simulink model "Casa"  (R2017a)
settings: Solver=ode45  StartTime=0.0  StopTime=5.0  RelTol=1e-3  EnableMultiTasking=on
libraries: simulink x3
settings Model: Creator=LAB1-8  LastModifiedBy=Oscar
settings DataIOCC: LimitDataPoints=on  SaveFormat=Array
settings OptimizationCC: LifeSpan=inf
settings DebuggingCC: UnderspecifiedInitializationDetection=Classic  MergeDetectMultiDrivingBlocksExec=none  SolverPrmCheckMsg=warning  SFUnexpectedBacktrackingDiag=warning  SFNoUnconditionalDefaultTransitionDiag=warning  SFExecutionAtInitializationDiag=none
settings HardwareCC: ProdBitPerPointer=32  ProdBitPerSizeT=32  ProdBitPerPtrDiffT=32  ProdLargestAtomicFloat=None  ProdIntDivRoundTo=Undefined  ProdEndianess=Unspecified  ProdWordSize=32  ProdHWDeviceType=32-bit Generic
settings ModelReferenceCC: PropagateSignalLabelsOutOfModel=off
settings GRTTargetCC: TargetLangStandard=C89/C90 (ANSI)  GeneratePreprocessorConditionals=Disable all
settings ConfigComp: CovMetricSettings=dw  CovHtmlReporting=on  CovSaveCumulativeToWorkspaceVar=on  CovSaveSingleToWorkspaceVar=on  CovExternalEMLEnable=off

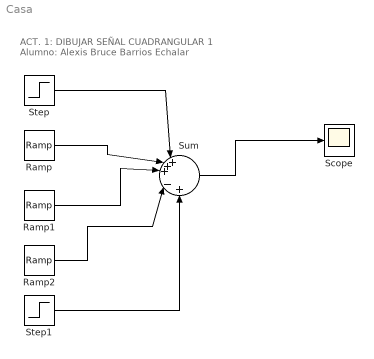
== system Casa ==
  note: ACT. 1: DIBUJAR SEÑAL CUADRANGULAR 1
      | Alumno: Alexis Bruce Barrios Echalar
  Ramp : simulink/Sources/Ramp  slope=1  start=1  X0=0
  Ramp1 : simulink/Sources/Ramp  slope=-2  start=2  X0=0
  Ramp2 : simulink/Sources/Ramp  slope=-1  start=3  X0=0
  Scope : Scope
  Step : Step  SampleTime=0
  Step1 : Step  Time=3  Before=1  After=0  SampleTime=0
  Sum : Sum  Inputs=|+++|-|+
  wires:
  Sum/1 -> Scope/1
  Step/1 -> Sum/1
  Ramp/1 -> Sum/2
  Ramp1/1 -> Sum/3
  Ramp2/1 -> Sum/4
  Step1/1 -> Sum/5
